simulink model "pwm_motor"  (R2017a)
settings: Solver=FixedStepAuto  StartTime=0.0  StopTime=tf  FixedStep=1e-6  RelTol=1e-3
values from neighbouring files (symbols this model uses):
  A = double(subs(A, symbs, vals))    [load_params.m]    (also in main.m)
  alpha = 0.5    [load_params.m]    (also in main.m)
  B = double(subs(B, symbs, vals))    [load_params.m]    (also in main.m)
  C = sysd.c    [load_discrete_pred_controller.m]    (also in load_params.m = double(subs(C, symbs, vals)); load_pwm_avg_pred_controller.m; main.m = double(subs(C, symbs, vals)))
  D = 0    [load_discrete_pred_controller.m]    (also in load_params.m = double(subs(D, symbs, vals)); main.m = double(subs(D, symbs, vals)))
  max_val = 2    [load_params.m]    (also in main.m = 12)
  min_val = 0    [load_params.m]    (also in main.m)
  T = 1e-3    (= 0.001)    [load_params.m]    (also in main.m)
  x0 = [0; 0; 0]    [main.m]    (also in sim_controlled_system.m = [0; 0]; sim_system.m)
settings Model: Creator=brunolnetto  LastModifiedBy=brunolnetto

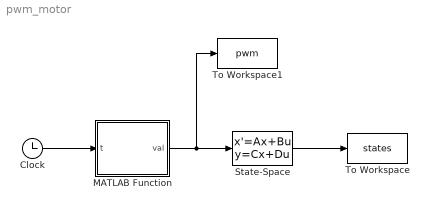
== system pwm_motor ==
  Clock : Clock
  MATLAB Function : MATLAB Function  TreatAsAtomicUnit=on
  State-Space : StateSpace  A=A  B=B  C=C  D=D  X0=x0
  To Workspace : ToWorkspace  VariableName=states  SaveFormat=Structure With Time  SampleTime=-1
  To Workspace1 : ToWorkspace  VariableName=pwm  SaveFormat=Structure With Time  SampleTime=-1
  wires:
  State-Space/1 -> To Workspace/1
  MATLAB Function/1(val) -> To Workspace1/1, State-Space/1
  Clock/1 -> MATLAB Function/1(t)

== matlab function pwm_motor/MATLAB Function ==
  data: t input; val output; max_val parameter; min_val parameter; alpha parameter; T parameter
function val = pwm_signal(t, max_val, min_val, alpha, T)
    persistent t0;
    if(isempty(t0))
        t0 = 0;
    end
    
    if(t == 0)
        t0 = 0;
    end

    if(t - t0 > T)
        t0 = t;
    end

    t_i = t - t0;
    
    if(t_i < alpha*T)
        val = max_val;
    else
        val = min_val;
    end
end
